simulink model "fkine_test"  (R2015a)
settings: Solver=ode45  StartTime=0.0  StopTime=10.0  RelTol=1e-3
values from neighbouring files (symbols this model uses):
  bL = 18.5    [runFirst.m]    (also in runFirst2.m = 20.5)
  bWb = 12.5    [runFirst.m]    (also in runFirst2.m = 14.5)
  bWs = 10.5    [runFirst.m]    (also in runFirst2.m = 12.5)
  d1 = 0    [runFirst.m]    (also in runFirst2.m)
  d2 = -4.61    [runFirst.m]    (also in runFirst2.m = 0)
  L1 = 3.64    [runFirst.m]    (also in runFirst2.m = 3.4)
  L2 = 5.72    [runFirst.m]    (also in runFirst2.m = 8.7)
  L3 = 12.46    [runFirst.m]    (also in runFirst2.m = 12.73)
libraries: roblocks x2
settings Model: Creator=340DANILOV  LastModifiedBy=340DANILOV

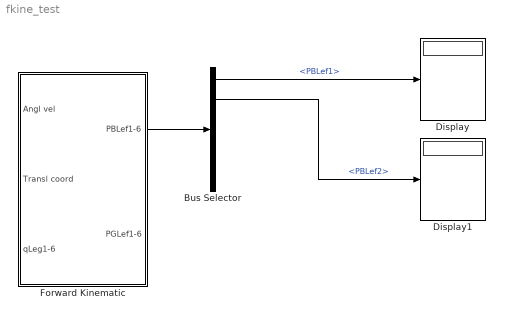
== system fkine_test ==
  Bus Selector : BusSelector  OutputSignals=PBLef1,PBLef2,PBLef3,PBLef4,PBLef5,PBLef6
  Display : Display
  Display1 : Display
  Forward Kinematic : Subsystem
  wires:
  Forward Kinematic/1(PBLef1-6) -> Bus Selector/1
  Bus Selector/1 -> Display/1  "<PBLef1>"
  Bus Selector/2 -> Display1/1  "<PBLef2>"

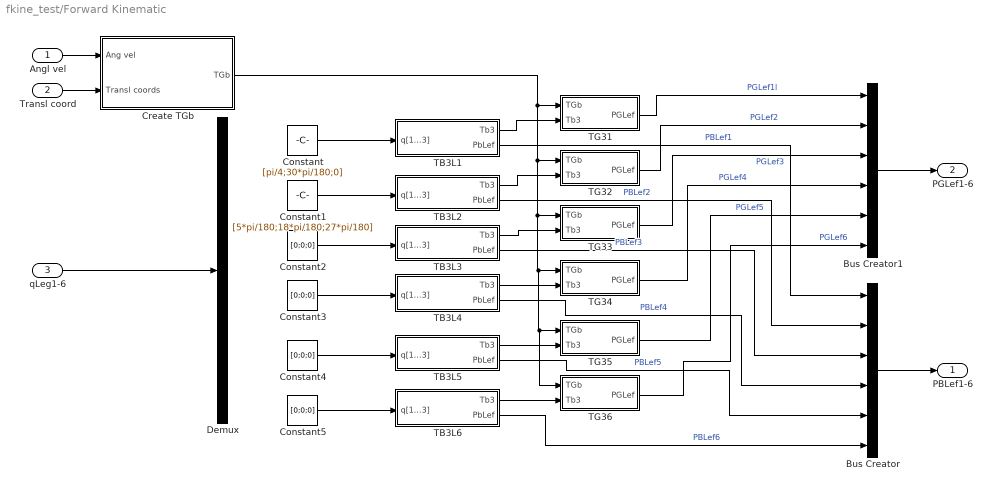
== system fkine_test/Forward Kinematic ==
  Angl vel : Inport
  Transl coord : Inport  Port=2
  qLeg1-6 : Inport  Port=3
  Bus Creator : BusCreator  Inputs=6
  Bus Creator1 : BusCreator  Inputs=6
  Constant : Constant  Value=[pi/4;30*pi/180;0]
  Constant1 : Constant  Value=[5*pi/180;18*pi/180;27*pi/180]
  Constant{2..5} (4 alike) : Constant  Value=[0;0;0]
  Create TGb : Subsystem
  Demux : Demux  Outputs=6
  TB3L1 : Subsystem
  TB3L2 : Subsystem
  TB3L3 : Subsystem
  TB3L4 : Subsystem
  TB3L5 : Subsystem
  TB3L6 : Subsystem
  TG31 : Subsystem
  TG32 : Subsystem
  TG33 : Subsystem
  TG34 : Subsystem
  TG35 : Subsystem
  TG36 : Subsystem
  PBLef1-6 : Outport
  PGLef1-6 : Outport  Port=2
  wires:
  TG34/1(PGLef) -> Bus Creator1/4  "PGLef4"
  TG36/1(PGLef) -> Bus Creator1/6  "PGLef6"
  TB3L5/1(Tb3) -> TG35/2(Tb3)
  qLeg1-6/1 -> Demux/1
  TB3L3/2(PbLef) -> Bus Creator/3  "PBLef3"
  Transl coord/1 -> Create TGb/2(Transl coords)
  Angl vel/1 -> Create TGb/1(Ang vel)
  Bus Creator1/1 -> PGLef1-6/1
  TG33/1(PGLef) -> Bus Creator1/3  "PGLef3"
  TB3L3/1(Tb3) -> TG33/2(Tb3)
  TB3L4/1(Tb3) -> TG34/2(Tb3)
  TG32/1(PGLef) -> Bus Creator1/2  "PGLef2"
  TB3L2/1(Tb3) -> TG32/2(Tb3)
  TB3L2/2(PbLef) -> Bus Creator/2  "PBLef2"
  TG31/1(PGLef) -> Bus Creator1/1  "PGLef1l"
  Create TGb/1(TGb) -> TG31/1(TGb), TG32/1(TGb), TG33/1(TGb), TG34/1(TGb), TG35/1(TGb), TG36/1(TGb)
  TB3L1/1(Tb3) -> TG31/2(Tb3)
  TB3L1/2(PbLef) -> Bus Creator/1  "PBLef1"
  TB3L6/2(PbLef) -> Bus Creator/6  "PBLef6"
  TG35/1(PGLef) -> Bus Creator1/5  "PGLef5"
  TB3L4/2(PbLef) -> Bus Creator/4  "PBLef4"
  TB3L5/2(PbLef) -> Bus Creator/5  "PBLef5"
  TB3L6/1(Tb3) -> TG36/2(Tb3)
  Bus Creator/1 -> PBLef1-6/1
  Constant/1 -> TB3L1/1(q[1...3])
  Constant1/1 -> TB3L2/1(q[1...3])
  Constant2/1 -> TB3L3/1(q[1...3])
  Constant3/1 -> TB3L4/1(q[1...3])
  Constant4/1 -> TB3L5/1(q[1...3])
  Constant5/1 -> TB3L6/1(q[1...3])

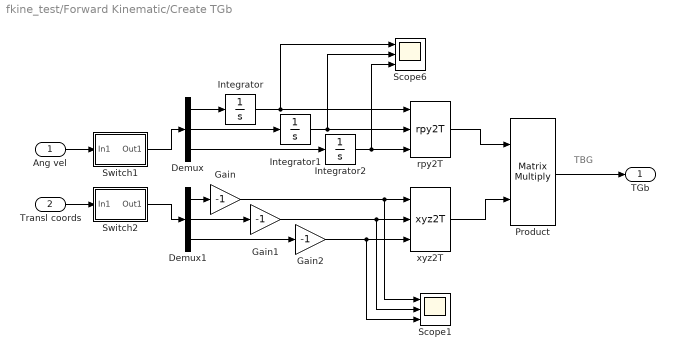
== system fkine_test/Forward Kinematic/Create TGb ==
  note: TBG
  Ang vel : Inport
  Transl coords : Inport  Port=2
  Demux : Demux  Outputs=3
  Demux1 : Demux  Outputs=3
  Gain : Gain  Gain=-1
  Gain1 : Gain  Gain=-1
  Gain2 : Gain  Gain=-1
  Integrator : Integrator
  Integrator1 : Integrator
  Integrator2 : Integrator
  Product : Product  Multiplication=Matrix(*)
  Scope1 : Scope  NumInputPorts=3
      settings: YMin=-15~-5~-5  YMax=20~5~5  SaveName=ScopeData38
  Scope6 : Scope  NumInputPorts=3
      settings: YMin=-15~-5~-5  YMax=20~5~5  SaveName=ScopeData48
  Switch1 : Subsystem
  Switch2 : Subsystem
  rpy2T : roblocks/Transform Conversion/rpy2T
      link override MATLAB Fcn: MATLABFcn=rpy2tr(u(1),u(2),u(3))
  xyz2T : roblocks/Transform Conversion/xyz2T
  TGb : Outport
  wires:
  Gain2/1 -> Scope1/3, xyz2T/3
  Gain1/1 -> Scope1/2, xyz2T/2
  Gain/1 -> xyz2T/1, Scope1/1
  Demux/1 -> Integrator/1
  Demux/2 -> Integrator1/1
  rpy2T/1 -> Product/1
  xyz2T/1 -> Product/2
  Product/1 -> TGb/1
  Demux/3 -> Integrator2/1
  Demux1/3 -> Gain2/1
  Demux1/2 -> Gain1/1
  Demux1/1 -> Gain/1
  Switch1/1(Out1) -> Demux/1
  Ang vel/1 -> Switch1/1(In1)
  Transl coords/1 -> Switch2/1(In1)
  Switch2/1(Out1) -> Demux1/1
  Integrator/1 -> rpy2T/1, Scope6/1
  Integrator2/1 -> rpy2T/3, Scope6/3
  Integrator1/1 -> rpy2T/2, Scope6/2

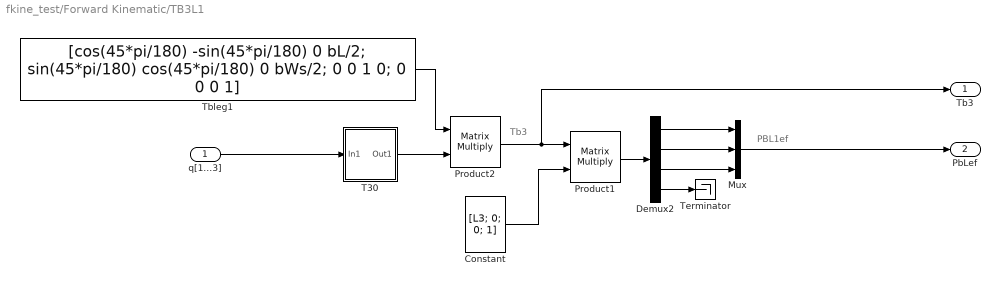
== system fkine_test/Forward Kinematic/TB3L1 ==
  note: PBL1ef
  note: Tb3
  q[1...3] : Inport
  Constant : Constant  Value=[L3; 0; 0; 1]  VectorParams1D=off
  Demux2 : Demux
  Mux : Mux  Inputs=3
  Product1 : Product  Multiplication=Matrix(*)
  Product2 : Product  Multiplication=Matrix(*)
  T30 : Subsystem
  Tbleg1 : Constant  Value=[cos(45*pi/180) -sin(45*pi/180) 0 bL/2; sin(45*pi/180) cos(45*pi/180) 0 bWs/2; 0 0 1 0; 0 0 0 1]  VectorParams1D=off
  Terminator : Terminator
  Tb3 : Outport
  PbLef : Outport  Port=2
  wires:
  Product2/1 -> Product1/1, Tb3/1
  Demux2/2 -> Mux/2
  Mux/1 -> PbLef/1
  Demux2/1 -> Mux/1
  Demux2/4 -> Terminator/1
  Product1/1 -> Demux2/1
  Demux2/3 -> Mux/3
  Tbleg1/1 -> Product2/1
  T30/1(Out1) -> Product2/2
  q[1...3]/1 -> T30/1(In1)
  Constant/1 -> Product1/2

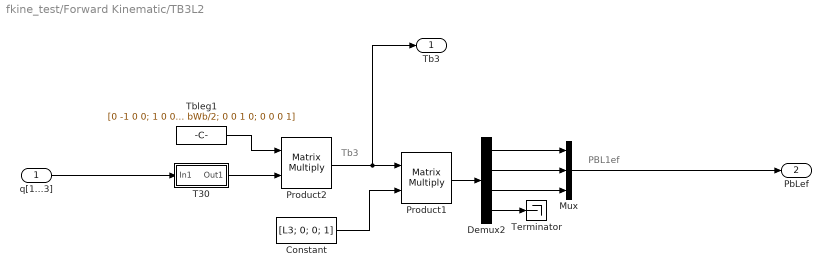
== system fkine_test/Forward Kinematic/TB3L2 ==
  note: Tb3
  note: PBL1ef
  q[1...3] : Inport
  Constant : Constant  Value=[L3; 0; 0; 1]  VectorParams1D=off
  Demux2 : Demux
  Mux : Mux  Inputs=3
  Product1 : Product  Multiplication=Matrix(*)
  Product2 : Product  Multiplication=Matrix(*)
  T30 : Subsystem
  Tbleg1 : Constant  Value=[0 -1 0 0; 1 0 0 bWb/2; 0 0 1 0; 0 0 0 1]  VectorParams1D=off
  Terminator : Terminator
  Tb3 : Outport
  PbLef : Outport  Port=2
  wires:
  Constant/1 -> Product1/2
  q[1...3]/1 -> T30/1(In1)
  T30/1(Out1) -> Product2/2
  Tbleg1/1 -> Product2/1
  Demux2/3 -> Mux/3
  Product1/1 -> Demux2/1
  Demux2/4 -> Terminator/1
  Demux2/1 -> Mux/1
  Mux/1 -> PbLef/1
  Demux2/2 -> Mux/2
  Product2/1 -> Tb3/1, Product1/1

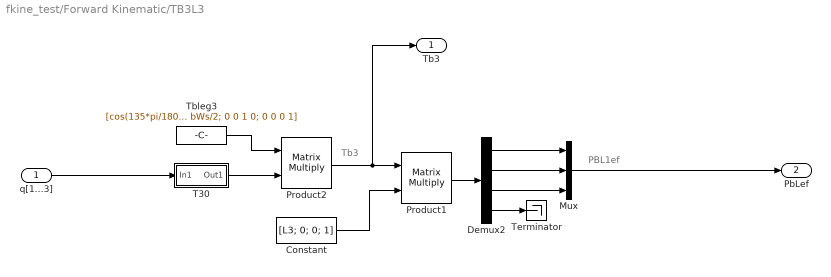
== system fkine_test/Forward Kinematic/TB3L3 ==
  note: PBL1ef
  note: Tb3
  q[1...3] : Inport
  Constant : Constant  Value=[L3; 0; 0; 1]  VectorParams1D=off
  Demux2 : Demux
  Mux : Mux  Inputs=3
  Product1 : Product  Multiplication=Matrix(*)
  Product2 : Product  Multiplication=Matrix(*)
  T30 : Subsystem
  Tbleg3 : Constant  Value=[cos(135*pi/180) -sin(135*pi/180) 0 -bL/2; sin(135*pi/180) cos(135*pi/180) 0 bWs/2; 0 0 1 0; 0 0 0 1]  VectorParams1D=off
  Terminator : Terminator
  Tb3 : Outport
  PbLef : Outport  Port=2
  wires:
  Product2/1 -> Product1/1, Tb3/1
  Demux2/2 -> Mux/2
  Mux/1 -> PbLef/1
  Demux2/1 -> Mux/1
  Demux2/4 -> Terminator/1
  Product1/1 -> Demux2/1
  Demux2/3 -> Mux/3
  Tbleg3/1 -> Product2/1
  T30/1(Out1) -> Product2/2
  q[1...3]/1 -> T30/1(In1)
  Constant/1 -> Product1/2

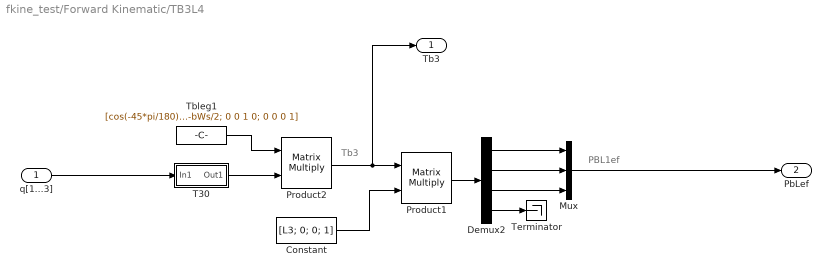
== system fkine_test/Forward Kinematic/TB3L4 ==
  note: Tb3
  note: PBL1ef
  q[1...3] : Inport
  Constant : Constant  Value=[L3; 0; 0; 1]  VectorParams1D=off
  Demux2 : Demux
  Mux : Mux  Inputs=3
  Product1 : Product  Multiplication=Matrix(*)
  Product2 : Product  Multiplication=Matrix(*)
  T30 : Subsystem
  Tbleg1 : Constant  Value=[cos(-45*pi/180) -sin(-45*pi/180) 0 bL/2; sin(-45*pi/180) cos(-45*pi/180) 0 -bWs/2; 0 0 1 0; 0 0 0 1]  VectorParams1D=off
  Terminator : Terminator
  Tb3 : Outport
  PbLef : Outport  Port=2
  wires:
  Constant/1 -> Product1/2
  q[1...3]/1 -> T30/1(In1)
  T30/1(Out1) -> Product2/2
  Tbleg1/1 -> Product2/1
  Demux2/3 -> Mux/3
  Product1/1 -> Demux2/1
  Demux2/4 -> Terminator/1
  Demux2/1 -> Mux/1
  Mux/1 -> PbLef/1
  Demux2/2 -> Mux/2
  Product2/1 -> Tb3/1, Product1/1

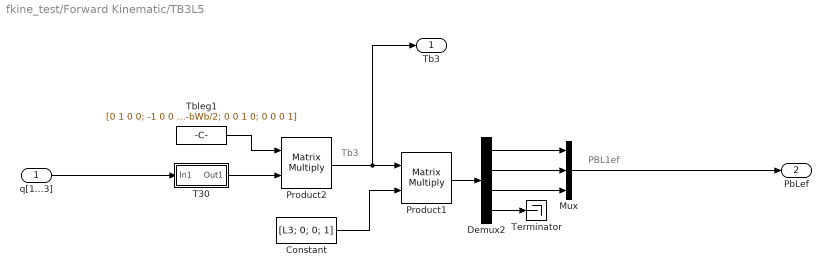
== system fkine_test/Forward Kinematic/TB3L5 ==
  note: PBL1ef
  note: Tb3
  q[1...3] : Inport
  Constant : Constant  Value=[L3; 0; 0; 1]  VectorParams1D=off
  Demux2 : Demux
  Mux : Mux  Inputs=3
  Product1 : Product  Multiplication=Matrix(*)
  Product2 : Product  Multiplication=Matrix(*)
  T30 : Subsystem
  Tbleg1 : Constant  Value=[0 1 0 0; -1 0 0 -bWb/2; 0 0 1 0; 0 0 0 1]  VectorParams1D=off
  Terminator : Terminator
  Tb3 : Outport
  PbLef : Outport  Port=2
  wires:
  Product2/1 -> Product1/1, Tb3/1
  Demux2/2 -> Mux/2
  Mux/1 -> PbLef/1
  Demux2/1 -> Mux/1
  Demux2/4 -> Terminator/1
  Product1/1 -> Demux2/1
  Demux2/3 -> Mux/3
  Tbleg1/1 -> Product2/1
  T30/1(Out1) -> Product2/2
  q[1...3]/1 -> T30/1(In1)
  Constant/1 -> Product1/2

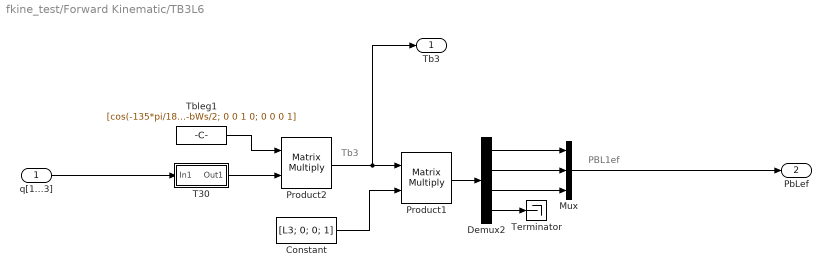
== system fkine_test/Forward Kinematic/TB3L6 ==
  note: PBL1ef
  note: Tb3
  q[1...3] : Inport
  Constant : Constant  Value=[L3; 0; 0; 1]  VectorParams1D=off
  Demux2 : Demux
  Mux : Mux  Inputs=3
  Product1 : Product  Multiplication=Matrix(*)
  Product2 : Product  Multiplication=Matrix(*)
  T30 : Subsystem
  Tbleg1 : Constant  Value=[cos(-135*pi/180) -sin(-135*pi/180) 0 -bL/2; sin(-135*pi/180) cos(-135*pi/180) 0 -bWs/2; 0 0 1 0; 0 0 0 1]  VectorParams1D=off
  Terminator : Terminator
  Tb3 : Outport
  PbLef : Outport  Port=2
  wires:
  Product2/1 -> Product1/1, Tb3/1
  Demux2/2 -> Mux/2
  Mux/1 -> PbLef/1
  Demux2/1 -> Mux/1
  Demux2/4 -> Terminator/1
  Product1/1 -> Demux2/1
  Demux2/3 -> Mux/3
  Tbleg1/1 -> Product2/1
  T30/1(Out1) -> Product2/2
  q[1...3]/1 -> T30/1(In1)
  Constant/1 -> Product1/2

== system fkine_test/Forward Kinematic/TG31 ==
  note: PGL1ef
  TGb : Inport
  Tb3 : Inport  Port=2
  Constant1 : Constant  Value=[0; L3; 0; 1]  VectorParams1D=off
  Demux1 : Demux
  Mux1 : Mux  Inputs=3
  Product3 : Product  Multiplication=Matrix(*)
  Product4 : Product  Multiplication=Matrix(*)
  Terminator1 : Terminator
  PGLef : Outport
  wires:
  Product3/1 -> Product4/1
  TGb/1 -> Product3/1
  Constant1/1 -> Product4/2
  Demux1/1 -> Mux1/1
  Product4/1 -> Demux1/1
  Mux1/1 -> PGLef/1
  Demux1/3 -> Mux1/3
  Demux1/4 -> Terminator1/1
  Demux1/2 -> Mux1/2
  Tb3/1 -> Product3/2

== system fkine_test/Forward Kinematic/TG32 ==
  note: PGL1ef
  TGb : Inport
  Tb3 : Inport  Port=2
  Constant1 : Constant  Value=[0; L3; 0; 1]  VectorParams1D=off
  Demux1 : Demux
  Mux1 : Mux  Inputs=3
  Product3 : Product  Multiplication=Matrix(*)
  Product4 : Product  Multiplication=Matrix(*)
  Terminator1 : Terminator
  PGLef : Outport
  wires:
  Tb3/1 -> Product3/2
  Demux1/2 -> Mux1/2
  Demux1/4 -> Terminator1/1
  Demux1/3 -> Mux1/3
  Mux1/1 -> PGLef/1
  Product4/1 -> Demux1/1
  Demux1/1 -> Mux1/1
  Constant1/1 -> Product4/2
  TGb/1 -> Product3/1
  Product3/1 -> Product4/1

== system fkine_test/Forward Kinematic/TG33 ==
  note: PGL1ef
  TGb : Inport
  Tb3 : Inport  Port=2
  Constant1 : Constant  Value=[0; L3; 0; 1]  VectorParams1D=off
  Demux1 : Demux
  Mux1 : Mux  Inputs=3
  Product3 : Product  Multiplication=Matrix(*)
  Product4 : Product  Multiplication=Matrix(*)
  Terminator1 : Terminator
  PGLef : Outport
  wires:
  Product3/1 -> Product4/1
  TGb/1 -> Product3/1
  Constant1/1 -> Product4/2
  Demux1/1 -> Mux1/1
  Product4/1 -> Demux1/1
  Mux1/1 -> PGLef/1
  Demux1/3 -> Mux1/3
  Demux1/4 -> Terminator1/1
  Demux1/2 -> Mux1/2
  Tb3/1 -> Product3/2

== system fkine_test/Forward Kinematic/TG34 ==
  note: PGL1ef
  TGb : Inport
  Tb3 : Inport  Port=2
  Constant1 : Constant  Value=[0; L3; 0; 1]  VectorParams1D=off
  Demux1 : Demux
  Mux1 : Mux  Inputs=3
  Product3 : Product  Multiplication=Matrix(*)
  Product4 : Product  Multiplication=Matrix(*)
  Terminator1 : Terminator
  PGLef : Outport
  wires:
  Tb3/1 -> Product3/2
  Demux1/2 -> Mux1/2
  Demux1/4 -> Terminator1/1
  Demux1/3 -> Mux1/3
  Mux1/1 -> PGLef/1
  Product4/1 -> Demux1/1
  Demux1/1 -> Mux1/1
  Constant1/1 -> Product4/2
  TGb/1 -> Product3/1
  Product3/1 -> Product4/1

== system fkine_test/Forward Kinematic/TG35 ==
  note: PGL1ef
  TGb : Inport
  Tb3 : Inport  Port=2
  Constant1 : Constant  Value=[0; L3; 0; 1]  VectorParams1D=off
  Demux1 : Demux
  Mux1 : Mux  Inputs=3
  Product3 : Product  Multiplication=Matrix(*)
  Product4 : Product  Multiplication=Matrix(*)
  Terminator1 : Terminator
  PGLef : Outport
  wires:
  Product3/1 -> Product4/1
  TGb/1 -> Product3/1
  Constant1/1 -> Product4/2
  Demux1/1 -> Mux1/1
  Product4/1 -> Demux1/1
  Mux1/1 -> PGLef/1
  Demux1/3 -> Mux1/3
  Demux1/4 -> Terminator1/1
  Demux1/2 -> Mux1/2
  Tb3/1 -> Product3/2

== system fkine_test/Forward Kinematic/TG36 ==
  note: PGL1ef
  TGb : Inport
  Tb3 : Inport  Port=2
  Constant1 : Constant  Value=[0; L3; 0; 1]  VectorParams1D=off
  Demux1 : Demux
  Mux1 : Mux  Inputs=3
  Product3 : Product  Multiplication=Matrix(*)
  Product4 : Product  Multiplication=Matrix(*)
  Terminator1 : Terminator
  PGLef : Outport
  wires:
  Product3/1 -> Product4/1
  TGb/1 -> Product3/1
  Constant1/1 -> Product4/2
  Demux1/1 -> Mux1/1
  Product4/1 -> Demux1/1
  Mux1/1 -> PGLef/1
  Demux1/3 -> Mux1/3
  Demux1/4 -> Terminator1/1
  Demux1/2 -> Mux1/2
  Tb3/1 -> Product3/2

== system fkine_test/Forward Kinematic/Create TGb/Switch1 ==
  In1 : Inport
  Constant : Constant  Value=0
  Switch : Switch  Threshold=0.5  SaturateOnIntegerOverflow=on  InputSameDT=on
  t <= 5 : Subsystem
  Out1 : Outport
  wires:
  Switch/1 -> Out1/1
  Constant/1 -> Switch/1
  t <= 5/1(t <= 1) -> Switch/2
  In1/1 -> Switch/3

== system fkine_test/Forward Kinematic/Create TGb/Switch2 ==
  In1 : Inport
  Constant1 : Constant  Value=0
  Switch1 : Switch  Threshold=0.5  SaturateOnIntegerOverflow=on  InputSameDT=on
  t <= 1 : Subsystem
  Out1 : Outport
  wires:
  Switch1/1 -> Out1/1
  In1/1 -> Switch1/3
  Constant1/1 -> Switch1/1
  t <= 1/1(t <= 1) -> Switch1/2

== system fkine_test/Forward Kinematic/TB3L1/T30 ==
  In1 : Inport
  Demux1 : Demux  Outputs=3
  Interpreted MATLAB Function : MATLABFcn  MATLABFcn=[cos(u) -sin(u) 0 0; sin(u) cos(u) 0 0; 0 0 1 d1; 0 0 0 1]  Output1D=off
  Interpreted MATLAB Function1 : MATLABFcn  MATLABFcn=[cos(u) -sin(u) 0 L1; 0 0 -1 0; sin(u) cos(u) 0 -abs(d2); 0 0 0 1]  Output1D=off
  Interpreted MATLAB Function2 : MATLABFcn  MATLABFcn=[cos(u+90*pi/180) -sin(u+90*pi/180) 0 L2; -sin(u+90*pi/180) -cos(u+90*pi/180) 0 0; 0 0 -1 0; 0 0 0 1]  Output1D=off
  Product : Product  Inputs=3  Multiplication=Matrix(*)
  Out1 : Outport
  wires:
  Demux1/1 -> Interpreted MATLAB Function/1
  In1/1 -> Demux1/1
  Product/1 -> Out1/1
  Demux1/2 -> Interpreted MATLAB Function1/1
  Demux1/3 -> Interpreted MATLAB Function2/1
  Interpreted MATLAB Function/1 -> Product/1
  Interpreted MATLAB Function1/1 -> Product/2
  Interpreted MATLAB Function2/1 -> Product/3

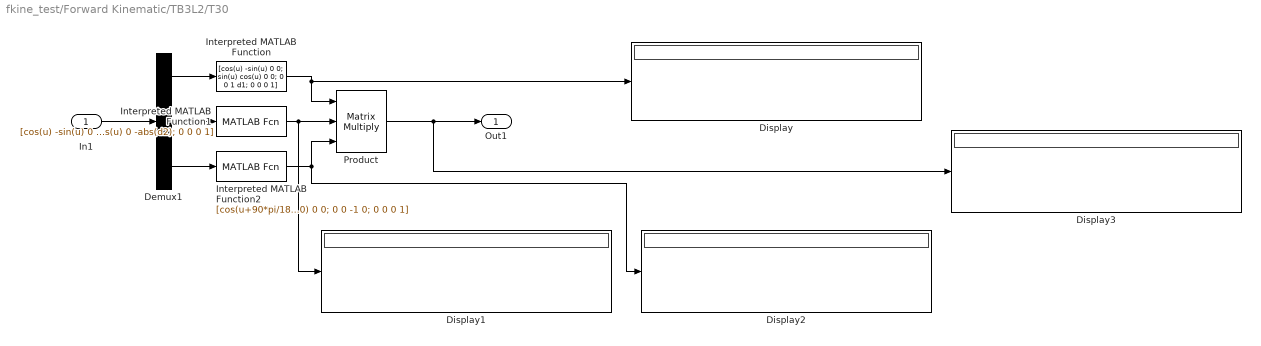
== system fkine_test/Forward Kinematic/TB3L2/T30 ==
  In1 : Inport
  Demux1 : Demux  Outputs=3
  Display{,1..3} (4 alike) : Display
  Interpreted MATLAB Function : MATLABFcn  MATLABFcn=[cos(u) -sin(u) 0 0; sin(u) cos(u) 0 0; 0 0 1 d1; 0 0 0 1]  Output1D=off
  Interpreted MATLAB Function1 : MATLABFcn  MATLABFcn=[cos(u) -sin(u) 0 L1; 0 0 -1 0; sin(u) cos(u) 0 -abs(d2); 0 0 0 1]  Output1D=off
  Interpreted MATLAB Function2 : MATLABFcn  MATLABFcn=[cos(u+90*pi/180) -sin(u+90*pi/180) 0 L2; -sin(u+90*pi/180) -cos(u+90*pi/180) 0 0; 0 0 -1 0; 0 0 0 1]  Output1D=off
  Product : Product  Inputs=3  Multiplication=Matrix(*)
  Out1 : Outport
  wires:
  Product/1 -> Out1/1, Display3/1
  Interpreted MATLAB Function/1 -> Product/1, Display/1
  Interpreted MATLAB Function2/1 -> Display2/1, Product/3
  Interpreted MATLAB Function1/1 -> Product/2, Display1/1
  Demux1/3 -> Interpreted MATLAB Function2/1
  Demux1/2 -> Interpreted MATLAB Function1/1
  In1/1 -> Demux1/1
  Demux1/1 -> Interpreted MATLAB Function/1

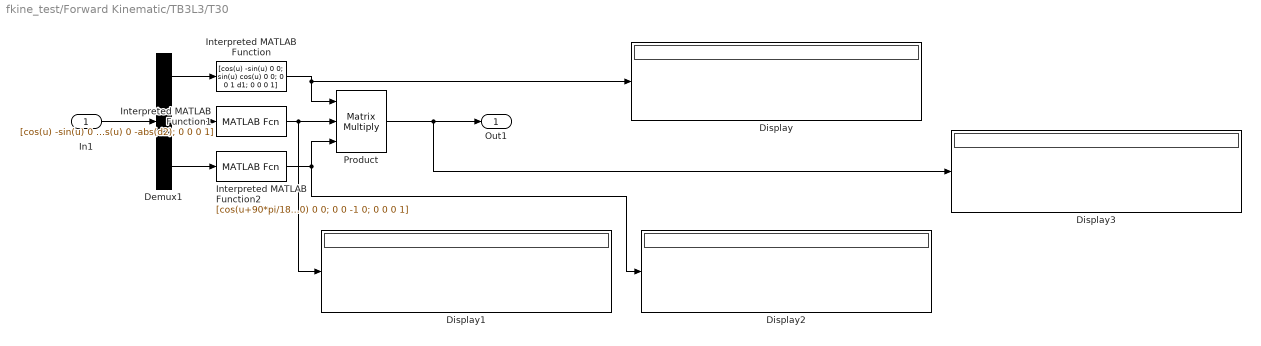
== system fkine_test/Forward Kinematic/TB3L3/T30 ==
  In1 : Inport
  Demux1 : Demux  Outputs=3
  Display{,1..3} (4 alike) : Display
  Interpreted MATLAB Function : MATLABFcn  MATLABFcn=[cos(u) -sin(u) 0 0; sin(u) cos(u) 0 0; 0 0 1 d1; 0 0 0 1]  Output1D=off
  Interpreted MATLAB Function1 : MATLABFcn  MATLABFcn=[cos(u) -sin(u) 0 L1; 0 0 -1 0; sin(u) cos(u) 0 -abs(d2); 0 0 0 1]  Output1D=off
  Interpreted MATLAB Function2 : MATLABFcn  MATLABFcn=[cos(u+90*pi/180) -sin(u+90*pi/180) 0 L2; -sin(u+90*pi/180) -cos(u+90*pi/180) 0 0; 0 0 -1 0; 0 0 0 1]  Output1D=off
  Product : Product  Inputs=3  Multiplication=Matrix(*)
  Out1 : Outport
  wires:
  Demux1/1 -> Interpreted MATLAB Function/1
  In1/1 -> Demux1/1
  Demux1/2 -> Interpreted MATLAB Function1/1
  Demux1/3 -> Interpreted MATLAB Function2/1
  Interpreted MATLAB Function1/1 -> Display1/1, Product/2
  Interpreted MATLAB Function2/1 -> Product/3, Display2/1
  Interpreted MATLAB Function/1 -> Display/1, Product/1
  Product/1 -> Display3/1, Out1/1

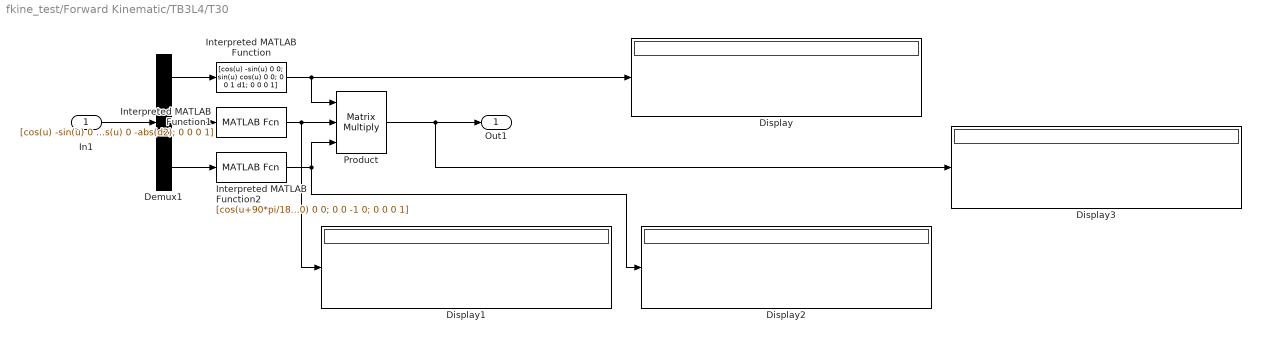
== system fkine_test/Forward Kinematic/TB3L4/T30 ==
  In1 : Inport
  Demux1 : Demux  Outputs=3
  Display{,1..3} (4 alike) : Display
  Interpreted MATLAB Function : MATLABFcn  MATLABFcn=[cos(u) -sin(u) 0 0; sin(u) cos(u) 0 0; 0 0 1 d1; 0 0 0 1]  Output1D=off
  Interpreted MATLAB Function1 : MATLABFcn  MATLABFcn=[cos(u) -sin(u) 0 L1; 0 0 -1 0; sin(u) cos(u) 0 -abs(d2); 0 0 0 1]  Output1D=off
  Interpreted MATLAB Function2 : MATLABFcn  MATLABFcn=[cos(u+90*pi/180) -sin(u+90*pi/180) 0 L2; -sin(u+90*pi/180) -cos(u+90*pi/180) 0 0; 0 0 -1 0; 0 0 0 1]  Output1D=off
  Product : Product  Inputs=3  Multiplication=Matrix(*)
  Out1 : Outport
  wires:
  Interpreted MATLAB Function2/1 -> Product/3, Display2/1
  Interpreted MATLAB Function1/1 -> Display1/1, Product/2
  Interpreted MATLAB Function/1 -> Product/1, Display/1
  Demux1/3 -> Interpreted MATLAB Function2/1
  Demux1/2 -> Interpreted MATLAB Function1/1
  Product/1 -> Display3/1, Out1/1
  In1/1 -> Demux1/1
  Demux1/1 -> Interpreted MATLAB Function/1

== system fkine_test/Forward Kinematic/TB3L5/T30 ==
  In1 : Inport
  Demux1 : Demux  Outputs=3
  Display{,1..3} (4 alike) : Display
  Interpreted MATLAB Function : MATLABFcn  MATLABFcn=[cos(u) -sin(u) 0 0; sin(u) cos(u) 0 0; 0 0 1 d1; 0 0 0 1]  Output1D=off
  Interpreted MATLAB Function1 : MATLABFcn  MATLABFcn=[cos(u) -sin(u) 0 L1; 0 0 -1 0; sin(u) cos(u) 0 -abs(d2); 0 0 0 1]  Output1D=off
  Interpreted MATLAB Function2 : MATLABFcn  MATLABFcn=[cos(u+90*pi/180) -sin(u+90*pi/180) 0 L2; -sin(u+90*pi/180) -cos(u+90*pi/180) 0 0; 0 0 -1 0; 0 0 0 1]  Output1D=off
  Product : Product  Inputs=3  Multiplication=Matrix(*)
  Out1 : Outport
  wires:
  Demux1/1 -> Interpreted MATLAB Function/1
  In1/1 -> Demux1/1
  Demux1/2 -> Interpreted MATLAB Function1/1
  Demux1/3 -> Interpreted MATLAB Function2/1
  Interpreted MATLAB Function1/1 -> Display1/1, Product/2
  Interpreted MATLAB Function2/1 -> Product/3, Display2/1
  Interpreted MATLAB Function/1 -> Display/1, Product/1
  Product/1 -> Display3/1, Out1/1

== system fkine_test/Forward Kinematic/TB3L6/T30 ==
  In1 : Inport
  Demux1 : Demux  Outputs=3
  Display{,1..3} (4 alike) : Display
  Interpreted MATLAB Function : MATLABFcn  MATLABFcn=[cos(u) -sin(u) 0 0; sin(u) cos(u) 0 0; 0 0 1 d1; 0 0 0 1]  Output1D=off
  Interpreted MATLAB Function1 : MATLABFcn  MATLABFcn=[cos(u) -sin(u) 0 L1; 0 0 -1 0; sin(u) cos(u) 0 -abs(d2); 0 0 0 1]  Output1D=off
  Interpreted MATLAB Function2 : MATLABFcn  MATLABFcn=[cos(u+90*pi/180) -sin(u+90*pi/180) 0 L2; -sin(u+90*pi/180) -cos(u+90*pi/180) 0 0; 0 0 -1 0; 0 0 0 1]  Output1D=off
  Product : Product  Inputs=3  Multiplication=Matrix(*)
  Out1 : Outport
  wires:
  Demux1/1 -> Interpreted MATLAB Function/1
  In1/1 -> Demux1/1
  Product/1 -> Out1/1, Display3/1
  Demux1/2 -> Interpreted MATLAB Function1/1
  Demux1/3 -> Interpreted MATLAB Function2/1
  Interpreted MATLAB Function/1 -> Display/1, Product/1
  Interpreted MATLAB Function1/1 -> Product/2, Display1/1
  Interpreted MATLAB Function2/1 -> Display2/1, Product/3

== system fkine_test/Forward Kinematic/Create TGb/Switch1/t <= 5 ==
  Clock : Clock
  Constant : Constant
  Relational Operator : RelationalOperator  Operator=<=  InputSameDT=on
  t <= 1 : Outport  InitialOutput=0
  wires:
  Constant/1 -> Relational Operator/2
  Clock/1 -> Relational Operator/1
  Relational Operator/1 -> t <= 1/1

== system fkine_test/Forward Kinematic/Create TGb/Switch2/t <= 1 ==
  Clock : Clock
  Constant : Constant
  Relational Operator : RelationalOperator  Operator=<=  InputSameDT=on
  t <= 1 : Outport  InitialOutput=0
  wires:
  Relational Operator/1 -> t <= 1/1
  Clock/1 -> Relational Operator/1
  Constant/1 -> Relational Operator/2
